simulink model "svpwmR2020a"  (Simulink 10.2)
settings: Solver=VariableStepAuto  StartTime=0.0  StopTime=0.05  RelTol=1e-3
libraries: powerlib x12, simulink x1
settings Model: Creator=Administrator  LastModifiedBy=Administrator
settings DataIOCC: SaveFormat=Dataset  SignalLoggingSaveFormat=Dataset
settings OptimizationCC: LifeSpan=auto
settings DebuggingCC: UnderspecifiedInitializationDetection=Simplified  MergeDetectMultiDrivingBlocksExec=error  FcnCallInpInsideContextMsg=error  SFUnexpectedBacktrackingDiag=error  SFNoUnconditionalDefaultTransitionDiag=error  SFExecutionAtInitializationDiag=warning
settings HardwareCC: ProdBitPerPointer=64  ProdBitPerSizeT=64  ProdBitPerPtrDiffT=64  ProdLargestAtomicFloat=Float  ProdIntDivRoundTo=Zero  ProdEndianess=LittleEndian  ProdWordSize=64  ProdHWDeviceType=Intel->x86-64 (Windows64)
settings ModelReferenceCC: PropagateSignalLabelsOutOfModel=on
settings GRTTargetCC: TargetLangStandard=C99 (ISO)  CombineOutputUpdateFcns=on  GRTInterface=off
settings ConfigComp: CovMetricSettings=dwe  CovSaveCumulativeToWorkspaceVar=off  CovSaveSingleToWorkspaceVar=off  CovExternalEMLEnable=on
settings SimscapeCC: SimscapeNormalizeSystem=off

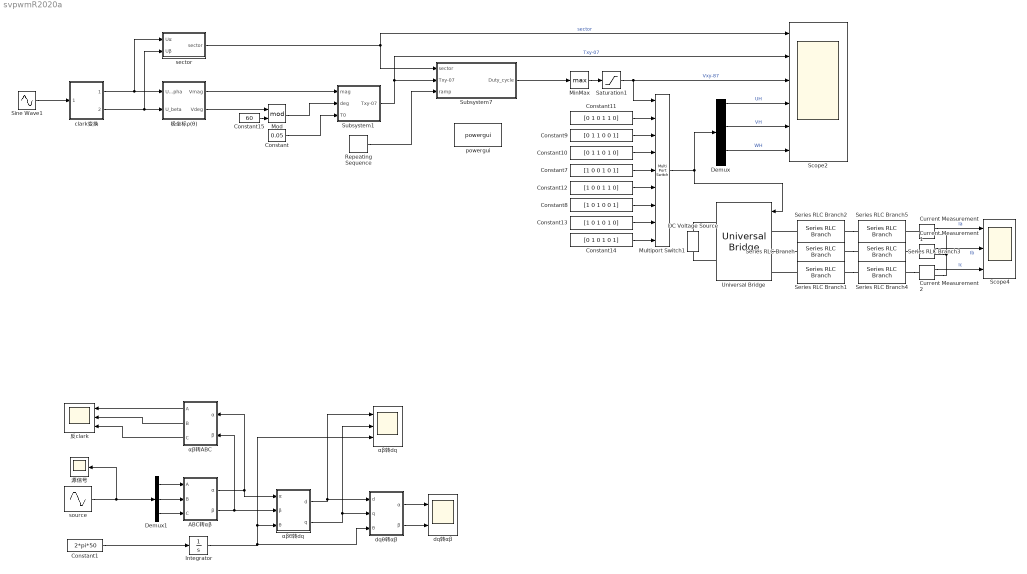
== system svpwmR2020a ==
  ABC转αβ : Subsystem
  Constant : Constant  Value=0.05
  Constant1 : Constant  Value=2*pi*50  SampleTime=1e-6
  Constant10 : Constant  Value=[0 1 1 0 1 0]  VectorParams1D=off  SampleTime=-1
  Constant11 : Constant  Value=[0 1 0 1 1 0]  VectorParams1D=off  SampleTime=-1
  Constant12 : Constant  Value=[1 0 0 1 1 0]  VectorParams1D=off  SampleTime=-1
  Constant13 : Constant  Value=[1 0 1 0 1 0]  VectorParams1D=off  SampleTime=-1
  Constant14 : Constant  Value=[0 1 0 1 0 1]  VectorParams1D=off  SampleTime=-1
  Constant15 : Constant  Value=60
  Constant7 : Constant  Value=[1 0 0 1 0 1]  VectorParams1D=off  SampleTime=-1
  Constant8 : Constant  Value=[1 0 1 0 0 1]  VectorParams1D=off  SampleTime=-1
  Constant9 : Constant  Value=[0 1 1 0 0 1]  VectorParams1D=off  SampleTime=-1
  Current Measurement : powerlib/Measurements/Current Measurement  PhasorSimulation=off  OutputType=Complex  PSBequivalent=0
  Current Measurement1 : powerlib/Measurements/Current Measurement  PhasorSimulation=off  OutputType=Complex  PSBequivalent=0
  Current Measurement2 : powerlib/Measurements/Current Measurement  PhasorSimulation=off  OutputType=Complex  PSBequivalent=0
  DC Voltage Source : powerlib/Electrical Sources/DC Voltage Source  Amplitude=100  Measurements=Voltage
  Demux : Demux  Outputs=6
  Demux1 : Demux  Outputs=3
  Integrator : Integrator
  MinMax : MinMax  Function=max
  Mod : Math  Operator=mod  SaturateOnIntegerOverflow=on
  Multiport Switch1 : MultiPortSwitch  Inputs=8
  Repeating Sequence : simulink/Sources/Repeating Sequence  rep_seq_t=[0 1e-4]  rep_seq_y=[0 1]
  Saturation1 : Saturate  UpperLimit=8  LowerLimit=1
  Scope2 : Scope  NumInputPorts=6
  Scope4 : Scope  NumInputPorts=3
  Series RLC Branch : powerlib/Elements/Series RLC Branch  LConnTagsString=__new0  RConnTagsString=__new0  BranchType=R  Resistance=2  Inductance=1e-3  SetiL0=off  InitialCurrent=0  Capacitance=1e-6  Setx0=off  InitialVoltage=0  Measurements=Branch current
  Series RLC Branch1 : powerlib/Elements/Series RLC Branch  LConnTagsString=__new0  RConnTagsString=__new0  BranchType=R  Resistance=2  Inductance=1e-3  SetiL0=off  InitialCurrent=0  Capacitance=1e-6  Setx0=off  InitialVoltage=0  Measurements=Branch current
  Series RLC Branch2 : powerlib/Elements/Series RLC Branch  LConnTagsString=__new0  RConnTagsString=__new0  BranchType=R  Resistance=2  Inductance=1e-3  SetiL0=off  InitialCurrent=0  Capacitance=1e-6  Setx0=off  InitialVoltage=0  Measurements=Branch current
  Series RLC Branch3 : powerlib/Elements/Series RLC Branch  LConnTagsString=__new0  RConnTagsString=__new0  BranchType=L  Resistance=2  Inductance=5e-3  SetiL0=off  InitialCurrent=0  Capacitance=1e-6  Setx0=off  InitialVoltage=0  Measurements=Branch current
  Series RLC Branch4 : powerlib/Elements/Series RLC Branch  LConnTagsString=__new0  RConnTagsString=__new0  BranchType=L  Resistance=2  Inductance=5e-3  SetiL0=off  InitialCurrent=0  Capacitance=1e-6  Setx0=off  InitialVoltage=0  Measurements=Branch current
  Series RLC Branch5 : powerlib/Elements/Series RLC Branch  LConnTagsString=__new0  RConnTagsString=__new0  BranchType=L  Resistance=2  Inductance=5e-3  SetiL0=off  InitialCurrent=0  Capacitance=1e-6  Setx0=off  InitialVoltage=0  Measurements=Branch current
  Sine Wave1 : Sin  Amplitude=0.5  Frequency=2*pi*50  Phase=[0 -2*pi/3 2*pi/3]  SampleTime=1e-6
  Subsystem1 : Subsystem
  Subsystem7 : Subsystem
  Universal Bridge : powerlib/Power Electronics/Universal Bridge  Arms=3  SnubberResistance=1e5  SnubberCapacitance=inf  Device=MOSFET / Diodes  Ron=1e-3  Lon=0  ForwardVoltages="[  50  50  ]"  ForwardVoltage=0  GTOparameters=[ 10e-6 , 20e-6 ]  IGBTparameters=[ 1e-6 , 2e-6 ]  Measurements=Device voltages  Measurements_2=None  converterType=Rectifier
  clark变换 : Subsystem
  dqθ转αβ : Subsystem
  dq转αβ : Scope  NumInputPorts=2
  powergui : powerlib/powergui  Priority=1  SimulationMode=Continuous  SampleTime=50e-6  frequency=60  Iterations=50  frequencyindice=0  Pbase=100e6  ErrMax=1e-4  UnitsV=kV  UnitsW=MW  buscounter=0  FunctionMessages=off  echomessages=off  EnableUseOfTLC=off  CurrentSourceSwitches=off  DisableSnubberDevices=off  DisableRonSwitches=off  DisableVfSwitches=off  DisplayEquations=off  AutomaticDiscreteSolvers=off  SolverType=Tustin/Backward Euler (TBE)  Interpol=off  ExternalGateDelay=off  methode=off  Ts=100  x0status=blocks  SPID=on  SwTol=0  HookPort=off  NonlinearTolerance=1e-4  nMaxIteration=100  ContinueOnMaxIteration=off  RestoreLinks=warning  ResistiveCurrentMeasurement=off  Frange=[0:2:500]  Ylog=off  Xlog=on  ShowGrid=off  save=off  variable=ZData  structure=0  ZoomFFT=off  StartTime=0.0  cycles=1  DisplayStyle=1  fundamental=60  FreqAxis=off  MaxFrequency=1000  frequencyindicesteady=1  RmsSteady=1  display=off
  sector : Subsystem
  source : Sin  Amplitude=100  Frequency=2*pi*50  Phase=[0 -2*pi/3 2*pi/3]  SampleTime=1e-6
  αβθ转dq : Subsystem
  αβ转ABC : Subsystem
  αβ转dq : Scope  NumInputPorts=3
  反clark : Scope  NumInputPorts=3
  极坐标ρ(θ) : Subsystem
  源信号 : Scope
  wires:
  Sine Wave1/1 -> clark变换/1(U_abc)
  极坐标ρ(θ)/2(Vdeg) -> Mod/1
  sector/1(sector) -> Scope2/1, Subsystem7/1(sector)  "sector"
  极坐标ρ(θ)/1("Vmag ") -> Subsystem1/1(mag)
  Constant/1 -> Subsystem1/3("T0 ")
  Subsystem1/1(Txy-07) -> Subsystem7/2(Txy-07), Scope2/2  "Txy-07"
  Repeating Sequence/1 -> Subsystem7/3(ramp)
  Subsystem7/1(Duty_cycle) -> MinMax/1
  MinMax/1 -> Saturation1/1
  Multiport Switch1/1 -> Demux/1, Universal Bridge/1
  Current Measurement/1 -> Scope4/1  "Ia"
  Current Measurement1/1 -> Scope4/2  "Ib"
  Current Measurement2/1 -> Scope4/3  "Ic"
  Demux/5 -> Scope2/6  "WH"
  Demux/3 -> Scope2/5  "VH"
  Demux/1 -> Scope2/4  "UH"
  Saturation1/1 -> Multiport Switch1/1, Scope2/3  "Vxy-87"
  Constant11/1 -> Multiport Switch1/2
  Constant9/1 -> Multiport Switch1/3
  Constant10/1 -> Multiport Switch1/4
  Constant7/1 -> Multiport Switch1/5
  Constant12/1 -> Multiport Switch1/6
  Constant8/1 -> Multiport Switch1/7
  Constant13/1 -> Multiport Switch1/8
  Constant14/1 -> Multiport Switch1/9
  clark变换/1(U_alpha) -> sector/1(Uα), 极坐标ρ(θ)/1("U_alpha ")
  clark变换/2(U_beta) -> sector/2(Uβ), 极坐标ρ(θ)/2(U_beta)
  Constant15/1 -> Mod/2
  Mod/1 -> Subsystem1/2(deg)
  Demux1/1 -> ABC转αβ/1(A)
  Demux1/3 -> ABC转αβ/3(C)
  Demux1/2 -> ABC转αβ/2(B)
  Constant1/1 -> Integrator/1
  source/1 -> Demux1/1, 源信号/1
  αβθ转dq/1(d) -> dqθ转αβ/1(d), αβ转dq/1
  Integrator/1 -> dqθ转αβ/3(θ), αβθ转dq/3(θ), αβ转dq/3
  αβθ转dq/2(q) -> αβ转dq/2, dqθ转αβ/2(q)
  αβ转ABC/2(B) -> 反clark/2
  αβ转ABC/1(A) -> 反clark/1
  αβ转ABC/3(C) -> 反clark/3
  ABC转αβ/2(β) -> αβ转ABC/2(β), αβθ转dq/2(β)
  ABC转αβ/1(α) -> αβ转ABC/1(α), αβθ转dq/1(α)
  dqθ转αβ/1(α) -> dq转αβ/1
  dqθ转αβ/2(β) -> dq转αβ/2
  connections:
  DC Voltage Source/RConn1 -- Universal Bridge/RConn1
  DC Voltage Source/LConn1 -- Universal Bridge/RConn2
  Series RLC Branch1/LConn1 -- Universal Bridge/LConn3
  Universal Bridge/LConn2 -- Series RLC Branch/LConn1
  Series RLC Branch2/LConn1 -- Universal Bridge/LConn1
  Series RLC Branch2/RConn1 -- Series RLC Branch5/LConn1
  Series RLC Branch/RConn1 -- Series RLC Branch3/LConn1
  Series RLC Branch1/RConn1 -- Series RLC Branch4/LConn1
  Current Measurement/LConn1 -- Series RLC Branch5/RConn1
  Series RLC Branch4/RConn1 -- Current Measurement2/LConn1
  Series RLC Branch3/RConn1 -- Current Measurement1/LConn1
  Current Measurement2/RConn1 -- Current Measurement1/RConn1 -- Current Measurement/RConn1

== system svpwmR2020a/ABC转αβ ==
  A : Inport
  B : Inport  Port=2
  C : Inport  Port=3
  Fcn : Fcn  Expr=2/3*(sqrt(3)/2*u(2)-sqrt(3)/2*u(3))
  Fcn1 : Fcn  Expr=2/3*(u(1)-0.5*u(2)-0.5*u(3))
  Mux : Mux  Inputs=3
  α : Outport
  β : Outport  Port=2
  wires:
  Mux/1 -> Fcn/1, Fcn1/1
  Fcn/1 -> β/1
  Fcn1/1 -> α/1
  A/1 -> Mux/1
  B/1 -> Mux/2
  C/1 -> Mux/3

== system svpwmR2020a/Subsystem1 ==
  mag : Inport
  deg : Inport  Port=2
  "T0 " : Inport  Port=3
  Mux : Mux
  duty-cycles : Subsystem
  Txy-07 : Outport
  wires:
  duty-cycles/2(Ty) -> Mux/2
  duty-cycles/4(T7) -> Mux/4
  duty-cycles/1(Tx) -> Mux/1
  deg/1 -> duty-cycles/2(deg)
  "T0 "/1 -> duty-cycles/3("T0 ")
  Mux/1 -> Txy-07/1
  duty-cycles/3(T0) -> Mux/3
  mag/1 -> duty-cycles/1(mag)

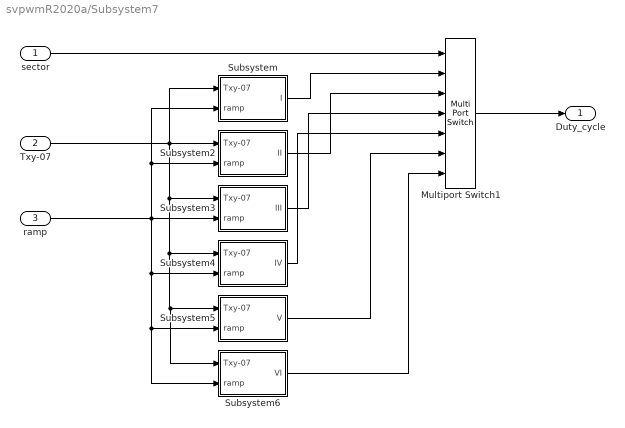
== system svpwmR2020a/Subsystem7 ==
  sector : Inport
  Txy-07 : Inport  Port=2
  ramp : Inport  Port=3
  Multiport Switch1 : MultiPortSwitch  Inputs=6
  Subsystem : Subsystem
  Subsystem2 : Subsystem
  Subsystem3 : Subsystem
  Subsystem4 : Subsystem
  Subsystem5 : Subsystem
  Subsystem6 : Subsystem
  Duty_cycle : Outport
  wires:
  Txy-07/1 -> Subsystem/1(Txy-07), Subsystem2/1(Txy-07), Subsystem3/1(Txy-07), Subsystem4/1(Txy-07), Subsystem6/1(Txy-07), Subsystem5/1(Txy-07)
  ramp/1 -> Subsystem3/2(ramp), Subsystem/2(ramp), Subsystem2/2(ramp), Subsystem5/2(ramp), Subsystem6/2(ramp), Subsystem4/2(ramp)
  Subsystem/1(I) -> Multiport Switch1/2
  Subsystem6/1(VI) -> Multiport Switch1/7
  Subsystem5/1(V) -> Multiport Switch1/6
  Subsystem3/1(III) -> Multiport Switch1/4
  Multiport Switch1/1 -> Duty_cycle/1
  Subsystem2/1(II) -> Multiport Switch1/3
  Subsystem4/1(IV) -> Multiport Switch1/5
  sector/1 -> Multiport Switch1/1

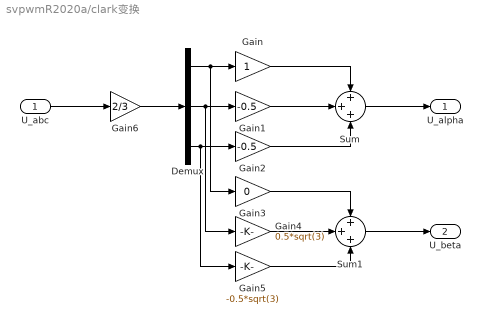
== system svpwmR2020a/clark变换 ==
  U_abc : Inport
  Demux : Demux  Outputs=3
  Gain : Gain
  Gain1 : Gain  Gain=-0.5
  Gain2 : Gain  Gain=-0.5
  Gain3 : Gain  Gain=0
  Gain4 : Gain  Gain=0.5*sqrt(3)
  Gain5 : Gain  Gain=-0.5*sqrt(3)
  Gain6 : Gain  Gain=2/3
  Sum : Sum  Inputs=+++
  Sum1 : Sum  Inputs=+++
  U_alpha : Outport
  U_beta : Outport  Port=2
  wires:
  Gain5/1 -> Sum1/3
  Gain4/1 -> Sum1/2
  Gain1/1 -> Sum/2
  Gain2/1 -> Sum/3
  Demux/1 -> Gain/1, Gain3/1
  Sum/1 -> U_alpha/1
  Sum1/1 -> U_beta/1
  Demux/3 -> Gain5/1, Gain2/1
  Gain/1 -> Sum/1
  Demux/2 -> Gain4/1, Gain1/1
  Gain3/1 -> Sum1/1
  U_abc/1 -> Gain6/1
  Gain6/1 -> Demux/1

== system svpwmR2020a/dqθ转αβ ==
  d : Inport
  q : Inport  Port=2
  θ : Inport  Port=3
  Fcn : Fcn  Expr=u(1)*sin(u(3))+u(2)*cos(u(3))
  Fcn1 : Fcn  Expr=u(1)*cos(u(3))-u(2)*sin(u(3))
  Mux : Mux  Inputs=3
  α : Outport
  β : Outport  Port=2
  wires:
  θ/1 -> Mux/3
  d/1 -> Mux/1
  Fcn1/1 -> α/1
  Fcn/1 -> β/1
  Mux/1 -> Fcn1/1, Fcn/1
  q/1 -> Mux/2

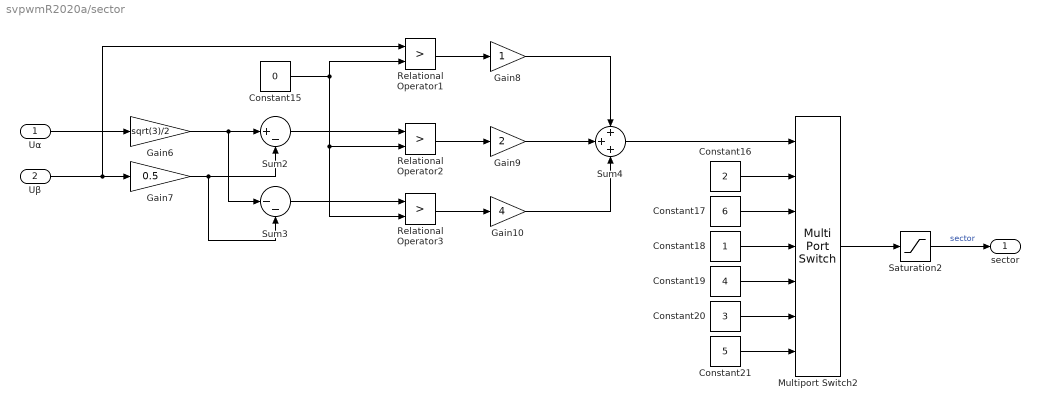
== system svpwmR2020a/sector ==
  Uα : Inport
  Uβ : Inport  Port=2
  Constant15 : Constant  Value=0
  Constant16 : Constant  Value=2
  Constant17 : Constant  Value=6
  Constant18 : Constant
  Constant19 : Constant  Value=4
  Constant20 : Constant  Value=3
  Constant21 : Constant  Value=5
  Gain10 : Gain  Gain=4
  Gain6 : Gain  Gain=sqrt(3)/2
  Gain7 : Gain  Gain=0.5
  Gain8 : Gain
  Gain9 : Gain  Gain=2
  Multiport Switch2 : MultiPortSwitch  Inputs=6
  Relational Operator1 : RelationalOperator  Operator=>  OutDataTypeStr=boolean  RndMeth=Simplest
  Relational Operator2 : RelationalOperator  Operator=>  OutDataTypeStr=boolean  RndMeth=Simplest
  Relational Operator3 : RelationalOperator  Operator=>  OutDataTypeStr=boolean  RndMeth=Simplest
  Saturation2 : Saturate  UpperLimit=6  LowerLimit=1
  Sum2 : Sum  Inputs=|+-
  Sum3 : Sum  Inputs=|--
  Sum4 : Sum  Inputs=+++
  sector : Outport
  wires:
  Relational Operator1/1 -> Gain8/1
  Sum3/1 -> Relational Operator3/1
  Gain6/1 -> Sum3/1, Sum2/1
  Constant15/1 -> Relational Operator1/2, Relational Operator3/2, Relational Operator2/2
  Gain9/1 -> Sum4/2
  Uβ/1 -> Relational Operator1/1, Gain7/1
  Relational Operator3/1 -> Gain10/1
  Relational Operator2/1 -> Gain9/1
  Constant17/1 -> Multiport Switch2/3
  Constant16/1 -> Multiport Switch2/2
  Constant21/1 -> Multiport Switch2/7
  Gain10/1 -> Sum4/3
  Gain7/1 -> Sum2/2, Sum3/2
  Sum2/1 -> Relational Operator2/1
  Uα/1 -> Gain6/1
  Constant18/1 -> Multiport Switch2/4
  Constant19/1 -> Multiport Switch2/5
  Constant20/1 -> Multiport Switch2/6
  Gain8/1 -> Sum4/1
  Sum4/1 -> Multiport Switch2/1
  Multiport Switch2/1 -> Saturation2/1
  Saturation2/1 -> sector/1  "sector"

== system svpwmR2020a/αβθ转dq ==
  α : Inport
  β : Inport  Port=2
  θ : Inport  Port=3
  Fcn : Fcn  Expr=-u(1)*sin(u(3))+u(2)*cos(u(3))
  Fcn1 : Fcn  Expr=u(1)*cos(u(3))+u(2)*sin(u(3))
  Gain : Gain
  Mux : Mux  Inputs=3
  d : Outport
  q : Outport  Port=2
  wires:
  θ/1 -> Mux/3
  β/1 -> Mux/2
  α/1 -> Mux/1
  Fcn1/1 -> d/1
  Mux/1 -> Fcn1/1, Fcn/1
  Fcn/1 -> Gain/1
  Gain/1 -> q/1

== system svpwmR2020a/αβ转ABC ==
  α : Inport
  β : Inport  Port=2
  Fcn : Fcn  Expr=-0.5*u(1)+sqrt(3)/2*u(2)
  Fcn1 : Fcn  Expr=u(1)
  Fcn2 : Fcn  Expr=-0.5*u(1)-sqrt(3)/2*u(2)
  Mux : Mux  Inputs=2
  A : Outport
  B : Outport  Port=2
  C : Outport  Port=3
  wires:
  β/1 -> Mux/2
  α/1 -> Mux/1
  Fcn1/1 -> A/1
  Fcn/1 -> B/1
  Mux/1 -> Fcn1/1, Fcn2/1, Fcn/1
  Fcn2/1 -> C/1

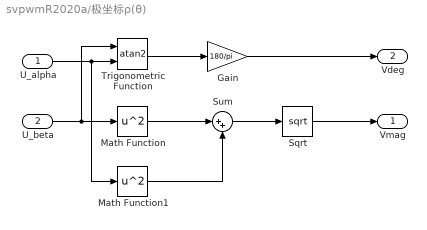
== system svpwmR2020a/极坐标ρ(θ) ==
  "U_alpha " : Inport
  U_beta : Inport  Port=2
  Gain : Gain  Gain=180/pi
  Math Function : Math  Operator=square  SignedPower=on  SaturateOnIntegerOverflow=on
  Math Function1 : Math  Operator=square  SignedPower=on  SaturateOnIntegerOverflow=on
  Sqrt : Sqrt  SaturateOnIntegerOverflow=on
  Sum : Sum  Inputs=|++
  Trigonometric Function : Trigonometry  Operator=atan2
  "Vmag " : Outport
  Vdeg : Outport  Port=2
  wires:
  "U_alpha "/1 -> Math Function1/1, Trigonometric Function/2
  U_beta/1 -> Trigonometric Function/1, Math Function/1
  Math Function/1 -> Sum/1
  Math Function1/1 -> Sum/2
  Sum/1 -> Sqrt/1
  Gain/1 -> Vdeg/1
  Trigonometric Function/1 -> Gain/1
  Sqrt/1 -> "Vmag "/1

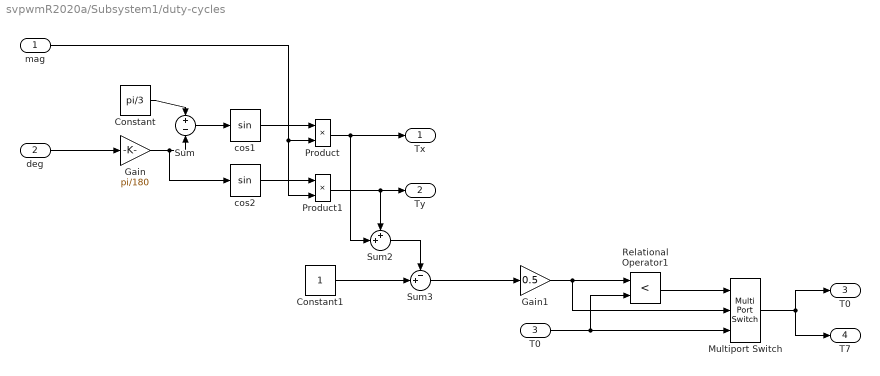
== system svpwmR2020a/Subsystem1/duty-cycles ==
  mag : Inport
  deg : Inport  Port=2
  "T0 " : Inport  Port=3
  Constant : Constant  Value=pi/3
  Constant1 : Constant
  Gain : Gain  Gain=pi/180
  Gain1 : Gain  Gain=0.5
  Multiport Switch : MultiPortSwitch  DataPortOrder=Zero-based contiguous  Inputs=2  zeroidx=on
  Product : Product
  Product1 : Product
  Relational Operator1 : RelationalOperator  Operator=<  OutDataTypeStr=boolean  RndMeth=Simplest
  Sum : Sum  Inputs=+|-
  Sum2 : Sum  Inputs=++|
  Sum3 : Sum  Inputs=-+|
  cos1 : Trigonometry
  cos2 : Trigonometry
  Tx : Outport
  Ty : Outport  Port=2
  T0 : Outport  Port=3
  T7 : Outport  Port=4
  wires:
  Gain/1 -> cos2/1, Sum/2
  cos1/1 -> Product/1
  Sum/1 -> cos1/1
  mag/1 -> Product1/2, Product/2
  deg/1 -> Gain/1
  Product1/1 -> Sum2/1, Ty/1
  Product/1 -> Sum2/2, Tx/1
  cos2/1 -> Product1/1
  Constant/1 -> Sum/1
  Sum2/1 -> Sum3/1
  Constant1/1 -> Sum3/2
  Sum3/1 -> Gain1/1
  Gain1/1 -> Multiport Switch/2, Relational Operator1/1
  "T0 "/1 -> Relational Operator1/2, Multiport Switch/3
  Relational Operator1/1 -> Multiport Switch/1
  Multiport Switch/1 -> T7/1, T0/1

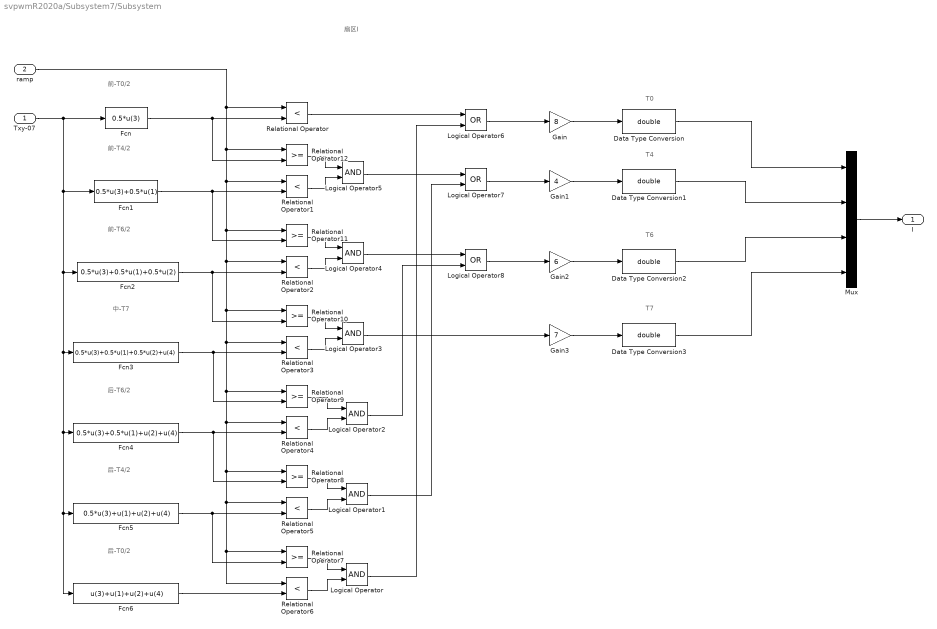
== system svpwmR2020a/Subsystem7/Subsystem ==
  note: 扇区I
  note: 前-T0/2
  note: 前-T4/2
  note: 前-T6/2
  note: 中-T7
  note: 后-T6/2
  note: 后-T4/2
  note: 后-T0/2
  note: T0
  note: T4
  note: T6
  note: T7
  Txy-07 : Inport
  ramp : Inport  Port=2
  Data Type Conversion{,1..3} (4 alike) : DataTypeConversion  OutDataTypeStr=double
  Fcn : Fcn  Expr=0.5*u(3)
  Fcn1 : Fcn  Expr=0.5*u(3)+0.5*u(1)
  Fcn2 : Fcn  Expr=0.5*u(3)+0.5*u(1)+0.5*u(2)
  Fcn3 : Fcn  Expr=0.5*u(3)+0.5*u(1)+0.5*u(2)+u(4)
  Fcn4 : Fcn  Expr=0.5*u(3)+0.5*u(1)+u(2)+u(4)
  Fcn5 : Fcn  Expr=0.5*u(3)+u(1)+u(2)+u(4)
  Fcn6 : Fcn  Expr=u(3)+u(1)+u(2)+u(4)
  Gain : Gain  Gain=8
  Gain1 : Gain  Gain=4
  Gain2 : Gain  Gain=6
  Gain3 : Gain  Gain=7
  Logical Operator{,1..5} (6 alike) : Logic  AllPortsSameDT=off  OutDataTypeStr=boolean
  Logical Operator6 : Logic  Operator=OR  AllPortsSameDT=off  OutDataTypeStr=boolean
  Logical Operator7 : Logic  Operator=OR  AllPortsSameDT=off  OutDataTypeStr=boolean
  Logical Operator8 : Logic  Operator=OR  AllPortsSameDT=off  OutDataTypeStr=boolean
  Mux : Mux
  Relational Operator{,1..6} (7 alike) : RelationalOperator  Operator=<  OutDataTypeStr=boolean  RndMeth=Simplest
  Relational Operator{7..12} (6 alike) : RelationalOperator  OutDataTypeStr=boolean  RndMeth=Simplest
  I : Outport
  wires:
  Txy-07/1 -> Fcn/1, Fcn1/1, Fcn2/1, Fcn6/1, Fcn5/1, Fcn4/1, Fcn3/1
  Fcn/1 -> Relational Operator12/2, Relational Operator/2
  Fcn1/1 -> Relational Operator11/2, Relational Operator1/2
  Fcn2/1 -> Relational Operator10/2, Relational Operator2/2
  Fcn3/1 -> Relational Operator9/2, Relational Operator3/2
  Fcn4/1 -> Relational Operator8/2, Relational Operator4/2
  Fcn6/1 -> Relational Operator6/2
  Fcn5/1 -> Relational Operator7/2, Relational Operator5/2
  Relational Operator7/1 -> Logical Operator/1
  Relational Operator6/1 -> Logical Operator/2
  Relational Operator12/1 -> Logical Operator5/1
  Relational Operator1/1 -> Logical Operator5/2
  Relational Operator11/1 -> Logical Operator4/1
  Relational Operator2/1 -> Logical Operator4/2
  Relational Operator10/1 -> Logical Operator3/1
  Relational Operator3/1 -> Logical Operator3/2
  Relational Operator9/1 -> Logical Operator2/1
  Relational Operator4/1 -> Logical Operator2/2
  Relational Operator8/1 -> Logical Operator1/1
  Relational Operator5/1 -> Logical Operator1/2
  ramp/1 -> Relational Operator12/1, Relational Operator11/1, Relational Operator10/1, Relational Operator9/1, Relational Operator8/1, Relational Operator7/1, Relational Operator6/1, Relational Operator5/1, Relational Operator4/1, Relational Operator3/1, Relational Operator2/1, Relational Operator1/1, Relational Operator/1
  Relational Operator/1 -> Logical Operator6/1
  Logical Operator/1 -> Logical Operator6/2
  Logical Operator5/1 -> Logical Operator7/1
  Logical Operator1/1 -> Logical Operator7/2
  Logical Operator4/1 -> Logical Operator8/1
  Logical Operator2/1 -> Logical Operator8/2
  Logical Operator6/1 -> Gain/1
  Logical Operator7/1 -> Gain1/1
  Logical Operator8/1 -> Gain2/1
  Logical Operator3/1 -> Gain3/1
  Gain3/1 -> Data Type Conversion3/1
  Gain2/1 -> Data Type Conversion2/1
  Gain1/1 -> Data Type Conversion1/1
  Gain/1 -> Data Type Conversion/1
  Data Type Conversion/1 -> Mux/1
  Data Type Conversion1/1 -> Mux/2
  Data Type Conversion2/1 -> Mux/3
  Data Type Conversion3/1 -> Mux/4
  Mux/1 -> I/1

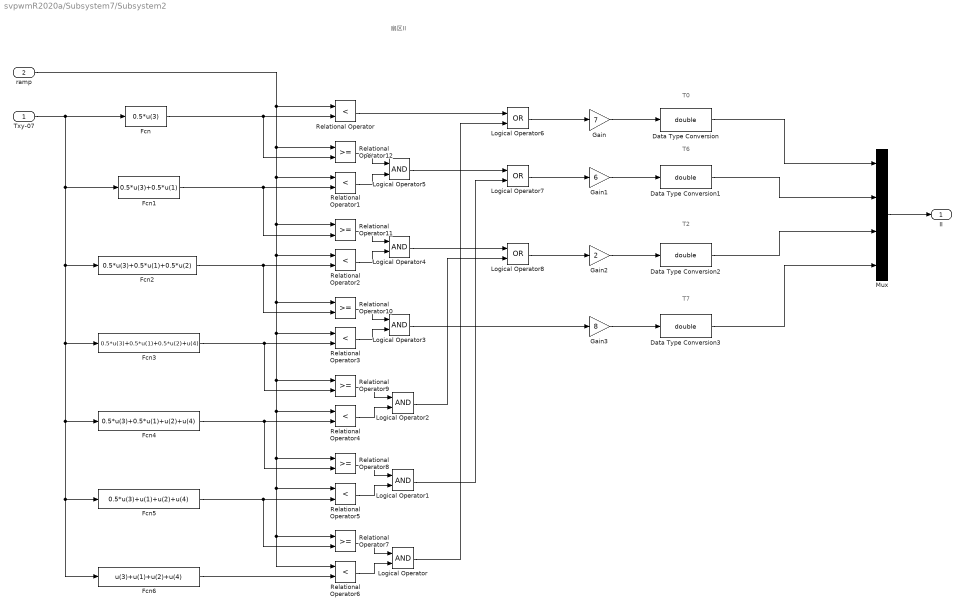
== system svpwmR2020a/Subsystem7/Subsystem2 ==
  note: T0
  note: 扇区II
  note: T2
  note: T7
  note: T6
  Txy-07 : Inport
  ramp : Inport  Port=2
  Data Type Conversion{,1..3} (4 alike) : DataTypeConversion  OutDataTypeStr=double
  Fcn : Fcn  Expr=0.5*u(3)
  Fcn1 : Fcn  Expr=0.5*u(3)+0.5*u(1)
  Fcn2 : Fcn  Expr=0.5*u(3)+0.5*u(1)+0.5*u(2)
  Fcn3 : Fcn  Expr=0.5*u(3)+0.5*u(1)+0.5*u(2)+u(4)
  Fcn4 : Fcn  Expr=0.5*u(3)+0.5*u(1)+u(2)+u(4)
  Fcn5 : Fcn  Expr=0.5*u(3)+u(1)+u(2)+u(4)
  Fcn6 : Fcn  Expr=u(3)+u(1)+u(2)+u(4)
  Gain : Gain  Gain=7
  Gain1 : Gain  Gain=6
  Gain2 : Gain  Gain=2
  Gain3 : Gain  Gain=8
  Logical Operator{,1..5} (6 alike) : Logic  AllPortsSameDT=off  OutDataTypeStr=boolean
  Logical Operator6 : Logic  Operator=OR  AllPortsSameDT=off  OutDataTypeStr=boolean
  Logical Operator7 : Logic  Operator=OR  AllPortsSameDT=off  OutDataTypeStr=boolean
  Logical Operator8 : Logic  Operator=OR  AllPortsSameDT=off  OutDataTypeStr=boolean
  Mux : Mux
  Relational Operator{,1..6} (7 alike) : RelationalOperator  Operator=<  OutDataTypeStr=boolean  RndMeth=Simplest
  Relational Operator{7..12} (6 alike) : RelationalOperator  OutDataTypeStr=boolean  RndMeth=Simplest
  II : Outport
  wires:
  Mux/1 -> II/1
  Data Type Conversion3/1 -> Mux/4
  Data Type Conversion2/1 -> Mux/3
  Data Type Conversion1/1 -> Mux/2
  Data Type Conversion/1 -> Mux/1
  Gain/1 -> Data Type Conversion/1
  Gain1/1 -> Data Type Conversion1/1
  Gain2/1 -> Data Type Conversion2/1
  Gain3/1 -> Data Type Conversion3/1
  Logical Operator3/1 -> Gain3/1
  Logical Operator8/1 -> Gain2/1
  Logical Operator7/1 -> Gain1/1
  Logical Operator6/1 -> Gain/1
  Logical Operator2/1 -> Logical Operator8/2
  Logical Operator4/1 -> Logical Operator8/1
  Logical Operator1/1 -> Logical Operator7/2
  Logical Operator5/1 -> Logical Operator7/1
  Logical Operator/1 -> Logical Operator6/2
  Relational Operator/1 -> Logical Operator6/1
  ramp/1 -> Relational Operator/1, Relational Operator1/1, Relational Operator2/1, Relational Operator3/1, Relational Operator4/1, Relational Operator5/1, Relational Operator6/1, Relational Operator7/1, Relational Operator8/1, Relational Operator9/1, Relational Operator10/1, Relational Operator11/1, Relational Operator12/1
  Relational Operator5/1 -> Logical Operator1/2
  Relational Operator8/1 -> Logical Operator1/1
  Relational Operator4/1 -> Logical Operator2/2
  Relational Operator9/1 -> Logical Operator2/1
  Relational Operator3/1 -> Logical Operator3/2
  Relational Operator10/1 -> Logical Operator3/1
  Relational Operator2/1 -> Logical Operator4/2
  Relational Operator11/1 -> Logical Operator4/1
  Relational Operator1/1 -> Logical Operator5/2
  Relational Operator12/1 -> Logical Operator5/1
  Relational Operator6/1 -> Logical Operator/2
  Relational Operator7/1 -> Logical Operator/1
  Fcn5/1 -> Relational Operator5/2, Relational Operator7/2
  Fcn6/1 -> Relational Operator6/2
  Fcn4/1 -> Relational Operator4/2, Relational Operator8/2
  Fcn3/1 -> Relational Operator3/2, Relational Operator9/2
  Fcn2/1 -> Relational Operator2/2, Relational Operator10/2
  Fcn1/1 -> Relational Operator1/2, Relational Operator11/2
  Fcn/1 -> Relational Operator/2, Relational Operator12/2
  Txy-07/1 -> Fcn/1, Fcn2/1, Fcn3/1, Fcn4/1, Fcn6/1, Fcn5/1, Fcn1/1

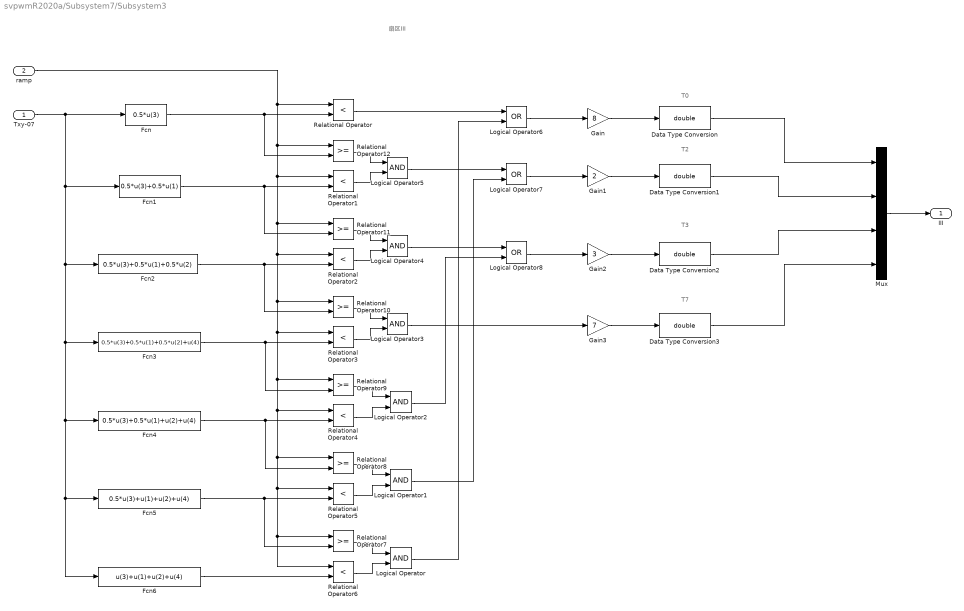
== system svpwmR2020a/Subsystem7/Subsystem3 ==
  note: T7
  note: 扇区III
  note: T0
  note: T2
  note: T3
  Txy-07 : Inport
  ramp : Inport  Port=2
  Data Type Conversion{,1..3} (4 alike) : DataTypeConversion  OutDataTypeStr=double
  Fcn : Fcn  Expr=0.5*u(3)
  Fcn1 : Fcn  Expr=0.5*u(3)+0.5*u(1)
  Fcn2 : Fcn  Expr=0.5*u(3)+0.5*u(1)+0.5*u(2)
  Fcn3 : Fcn  Expr=0.5*u(3)+0.5*u(1)+0.5*u(2)+u(4)
  Fcn4 : Fcn  Expr=0.5*u(3)+0.5*u(1)+u(2)+u(4)
  Fcn5 : Fcn  Expr=0.5*u(3)+u(1)+u(2)+u(4)
  Fcn6 : Fcn  Expr=u(3)+u(1)+u(2)+u(4)
  Gain : Gain  Gain=8
  Gain1 : Gain  Gain=2
  Gain2 : Gain  Gain=3
  Gain3 : Gain  Gain=7
  Logical Operator{,1..5} (6 alike) : Logic  AllPortsSameDT=off  OutDataTypeStr=boolean
  Logical Operator6 : Logic  Operator=OR  AllPortsSameDT=off  OutDataTypeStr=boolean
  Logical Operator7 : Logic  Operator=OR  AllPortsSameDT=off  OutDataTypeStr=boolean
  Logical Operator8 : Logic  Operator=OR  AllPortsSameDT=off  OutDataTypeStr=boolean
  Mux : Mux
  Relational Operator{,1..6} (7 alike) : RelationalOperator  Operator=<  OutDataTypeStr=boolean  RndMeth=Simplest
  Relational Operator{7..12} (6 alike) : RelationalOperator  OutDataTypeStr=boolean  RndMeth=Simplest
  III : Outport
  wires:
  Relational Operator7/1 -> Logical Operator/1
  Relational Operator6/1 -> Logical Operator/2
  Relational Operator12/1 -> Logical Operator5/1
  Relational Operator1/1 -> Logical Operator5/2
  Relational Operator11/1 -> Logical Operator4/1
  Relational Operator2/1 -> Logical Operator4/2
  Relational Operator10/1 -> Logical Operator3/1
  Relational Operator3/1 -> Logical Operator3/2
  Relational Operator9/1 -> Logical Operator2/1
  Relational Operator4/1 -> Logical Operator2/2
  Relational Operator8/1 -> Logical Operator1/1
  Relational Operator5/1 -> Logical Operator1/2
  Relational Operator/1 -> Logical Operator6/1
  Logical Operator/1 -> Logical Operator6/2
  Logical Operator5/1 -> Logical Operator7/1
  Logical Operator1/1 -> Logical Operator7/2
  Logical Operator4/1 -> Logical Operator8/1
  Logical Operator2/1 -> Logical Operator8/2
  Logical Operator6/1 -> Gain/1
  Logical Operator7/1 -> Gain1/1
  Logical Operator8/1 -> Gain2/1
  Logical Operator3/1 -> Gain3/1
  Gain3/1 -> Data Type Conversion3/1
  Gain2/1 -> Data Type Conversion2/1
  Gain1/1 -> Data Type Conversion1/1
  Gain/1 -> Data Type Conversion/1
  Data Type Conversion/1 -> Mux/1
  Data Type Conversion1/1 -> Mux/2
  Data Type Conversion2/1 -> Mux/3
  Data Type Conversion3/1 -> Mux/4
  Mux/1 -> III/1
  Fcn1/1 -> Relational Operator1/2, Relational Operator11/2
  Fcn3/1 -> Relational Operator9/2, Relational Operator3/2
  ramp/1 -> Relational Operator/1, Relational Operator12/1, Relational Operator1/1, Relational Operator11/1, Relational Operator2/1, Relational Operator10/1, Relational Operator3/1, Relational Operator9/1, Relational Operator4/1, Relational Operator8/1, Relational Operator5/1, Relational Operator7/1, Relational Operator6/1
  Fcn6/1 -> Relational Operator6/2
  Txy-07/1 -> Fcn/1, Fcn2/1, Fcn3/1, Fcn4/1, Fcn6/1, Fcn5/1, Fcn1/1
  Fcn2/1 -> Relational Operator10/2, Relational Operator2/2
  Fcn5/1 -> Relational Operator7/2, Relational Operator5/2
  Fcn4/1 -> Relational Operator4/2, Relational Operator8/2
  Fcn/1 -> Relational Operator12/2, Relational Operator/2

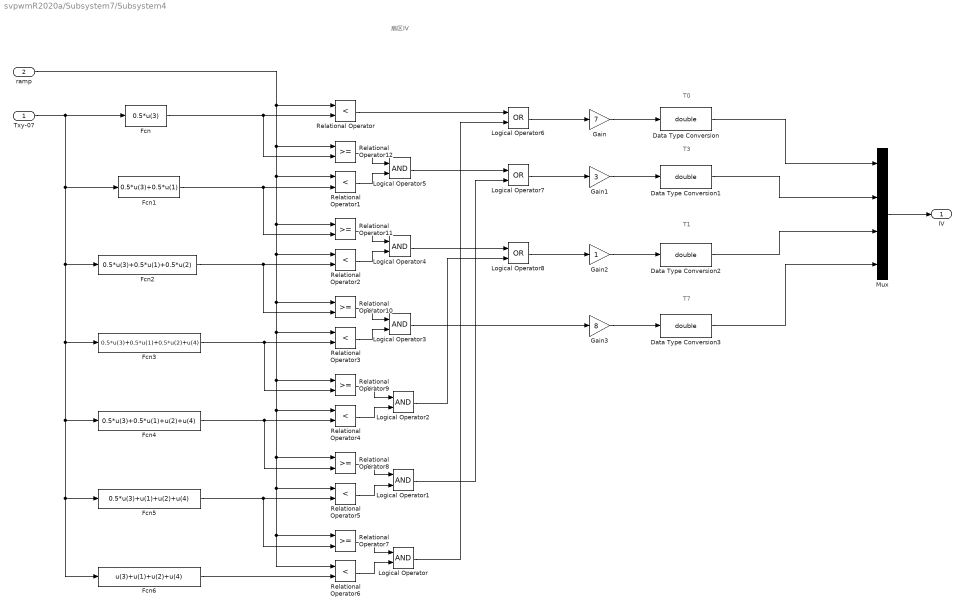
== system svpwmR2020a/Subsystem7/Subsystem4 ==
  note: T7
  note: 扇区IV
  note: T0
  note: T3
  note: T1
  Txy-07 : Inport
  ramp : Inport  Port=2
  Data Type Conversion{,1..3} (4 alike) : DataTypeConversion  OutDataTypeStr=double
  Fcn : Fcn  Expr=0.5*u(3)
  Fcn1 : Fcn  Expr=0.5*u(3)+0.5*u(1)
  Fcn2 : Fcn  Expr=0.5*u(3)+0.5*u(1)+0.5*u(2)
  Fcn3 : Fcn  Expr=0.5*u(3)+0.5*u(1)+0.5*u(2)+u(4)
  Fcn4 : Fcn  Expr=0.5*u(3)+0.5*u(1)+u(2)+u(4)
  Fcn5 : Fcn  Expr=0.5*u(3)+u(1)+u(2)+u(4)
  Fcn6 : Fcn  Expr=u(3)+u(1)+u(2)+u(4)
  Gain : Gain  Gain=7
  Gain1 : Gain  Gain=3
  Gain2 : Gain
  Gain3 : Gain  Gain=8
  Logical Operator{,1..5} (6 alike) : Logic  AllPortsSameDT=off  OutDataTypeStr=boolean
  Logical Operator6 : Logic  Operator=OR  AllPortsSameDT=off  OutDataTypeStr=boolean
  Logical Operator7 : Logic  Operator=OR  AllPortsSameDT=off  OutDataTypeStr=boolean
  Logical Operator8 : Logic  Operator=OR  AllPortsSameDT=off  OutDataTypeStr=boolean
  Mux : Mux
  Relational Operator{,1..6} (7 alike) : RelationalOperator  Operator=<  OutDataTypeStr=boolean  RndMeth=Simplest
  Relational Operator{7..12} (6 alike) : RelationalOperator  OutDataTypeStr=boolean  RndMeth=Simplest
  IV : Outport
  wires:
  Mux/1 -> IV/1
  Data Type Conversion3/1 -> Mux/4
  Data Type Conversion2/1 -> Mux/3
  Data Type Conversion1/1 -> Mux/2
  Data Type Conversion/1 -> Mux/1
  Gain/1 -> Data Type Conversion/1
  Gain1/1 -> Data Type Conversion1/1
  Gain2/1 -> Data Type Conversion2/1
  Gain3/1 -> Data Type Conversion3/1
  Logical Operator3/1 -> Gain3/1
  Logical Operator8/1 -> Gain2/1
  Logical Operator7/1 -> Gain1/1
  Logical Operator6/1 -> Gain/1
  Logical Operator2/1 -> Logical Operator8/2
  Logical Operator4/1 -> Logical Operator8/1
  Logical Operator1/1 -> Logical Operator7/2
  Logical Operator5/1 -> Logical Operator7/1
  Logical Operator/1 -> Logical Operator6/2
  Relational Operator/1 -> Logical Operator6/1
  Relational Operator5/1 -> Logical Operator1/2
  Relational Operator8/1 -> Logical Operator1/1
  Relational Operator4/1 -> Logical Operator2/2
  Relational Operator9/1 -> Logical Operator2/1
  Relational Operator3/1 -> Logical Operator3/2
  Relational Operator10/1 -> Logical Operator3/1
  Relational Operator2/1 -> Logical Operator4/2
  Relational Operator11/1 -> Logical Operator4/1
  Relational Operator1/1 -> Logical Operator5/2
  Relational Operator12/1 -> Logical Operator5/1
  Relational Operator6/1 -> Logical Operator/2
  Relational Operator7/1 -> Logical Operator/1
  Fcn1/1 -> Relational Operator11/2, Relational Operator1/2
  Fcn3/1 -> Relational Operator3/2, Relational Operator9/2
  ramp/1 -> Relational Operator/1, Relational Operator12/1, Relational Operator1/1, Relational Operator11/1, Relational Operator2/1, Relational Operator10/1, Relational Operator3/1, Relational Operator9/1, Relational Operator4/1, Relational Operator8/1, Relational Operator5/1, Relational Operator6/1, Relational Operator7/1
  Fcn6/1 -> Relational Operator6/2
  Txy-07/1 -> Fcn/1, Fcn2/1, Fcn3/1, Fcn4/1, Fcn6/1, Fcn5/1, Fcn1/1
  Fcn2/1 -> Relational Operator10/2, Relational Operator2/2
  Fcn5/1 -> Relational Operator5/2, Relational Operator7/2
  Fcn4/1 -> Relational Operator4/2, Relational Operator8/2
  Fcn/1 -> Relational Operator12/2, Relational Operator/2

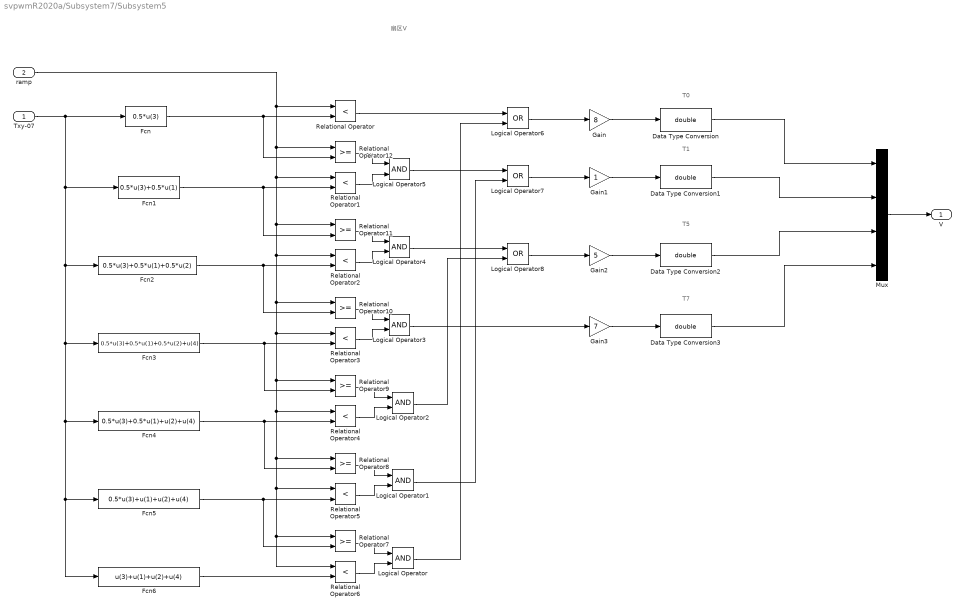
== system svpwmR2020a/Subsystem7/Subsystem5 ==
  note: T7
  note: 扇区V
  note: T0
  note: T1
  note: T5
  Txy-07 : Inport
  ramp : Inport  Port=2
  Data Type Conversion{,1..3} (4 alike) : DataTypeConversion  OutDataTypeStr=double
  Fcn : Fcn  Expr=0.5*u(3)
  Fcn1 : Fcn  Expr=0.5*u(3)+0.5*u(1)
  Fcn2 : Fcn  Expr=0.5*u(3)+0.5*u(1)+0.5*u(2)
  Fcn3 : Fcn  Expr=0.5*u(3)+0.5*u(1)+0.5*u(2)+u(4)
  Fcn4 : Fcn  Expr=0.5*u(3)+0.5*u(1)+u(2)+u(4)
  Fcn5 : Fcn  Expr=0.5*u(3)+u(1)+u(2)+u(4)
  Fcn6 : Fcn  Expr=u(3)+u(1)+u(2)+u(4)
  Gain : Gain  Gain=8
  Gain1 : Gain
  Gain2 : Gain  Gain=5
  Gain3 : Gain  Gain=7
  Logical Operator{,1..5} (6 alike) : Logic  AllPortsSameDT=off  OutDataTypeStr=boolean
  Logical Operator6 : Logic  Operator=OR  AllPortsSameDT=off  OutDataTypeStr=boolean
  Logical Operator7 : Logic  Operator=OR  AllPortsSameDT=off  OutDataTypeStr=boolean
  Logical Operator8 : Logic  Operator=OR  AllPortsSameDT=off  OutDataTypeStr=boolean
  Mux : Mux
  Relational Operator{,1..6} (7 alike) : RelationalOperator  Operator=<  OutDataTypeStr=boolean  RndMeth=Simplest
  Relational Operator{7..12} (6 alike) : RelationalOperator  OutDataTypeStr=boolean  RndMeth=Simplest
  V : Outport
  wires:
  Relational Operator7/1 -> Logical Operator/1
  Relational Operator6/1 -> Logical Operator/2
  Relational Operator12/1 -> Logical Operator5/1
  Relational Operator1/1 -> Logical Operator5/2
  Relational Operator11/1 -> Logical Operator4/1
  Relational Operator2/1 -> Logical Operator4/2
  Relational Operator10/1 -> Logical Operator3/1
  Relational Operator3/1 -> Logical Operator3/2
  Relational Operator9/1 -> Logical Operator2/1
  Relational Operator4/1 -> Logical Operator2/2
  Relational Operator8/1 -> Logical Operator1/1
  Relational Operator5/1 -> Logical Operator1/2
  Relational Operator/1 -> Logical Operator6/1
  Logical Operator/1 -> Logical Operator6/2
  Logical Operator5/1 -> Logical Operator7/1
  Logical Operator1/1 -> Logical Operator7/2
  Logical Operator4/1 -> Logical Operator8/1
  Logical Operator2/1 -> Logical Operator8/2
  Logical Operator6/1 -> Gain/1
  Logical Operator7/1 -> Gain1/1
  Logical Operator8/1 -> Gain2/1
  Logical Operator3/1 -> Gain3/1
  Gain3/1 -> Data Type Conversion3/1
  Gain2/1 -> Data Type Conversion2/1
  Gain1/1 -> Data Type Conversion1/1
  Gain/1 -> Data Type Conversion/1
  Data Type Conversion/1 -> Mux/1
  Data Type Conversion1/1 -> Mux/2
  Data Type Conversion2/1 -> Mux/3
  Data Type Conversion3/1 -> Mux/4
  Mux/1 -> V/1
  Fcn1/1 -> Relational Operator1/2, Relational Operator11/2
  Fcn3/1 -> Relational Operator9/2, Relational Operator3/2
  ramp/1 -> Relational Operator/1, Relational Operator12/1, Relational Operator1/1, Relational Operator11/1, Relational Operator2/1, Relational Operator10/1, Relational Operator3/1, Relational Operator9/1, Relational Operator4/1, Relational Operator8/1, Relational Operator5/1, Relational Operator7/1, Relational Operator6/1
  Fcn6/1 -> Relational Operator6/2
  Txy-07/1 -> Fcn/1, Fcn2/1, Fcn3/1, Fcn4/1, Fcn6/1, Fcn5/1, Fcn1/1
  Fcn2/1 -> Relational Operator10/2, Relational Operator2/2
  Fcn5/1 -> Relational Operator5/2, Relational Operator7/2
  Fcn4/1 -> Relational Operator8/2, Relational Operator4/2
  Fcn/1 -> Relational Operator12/2, Relational Operator/2

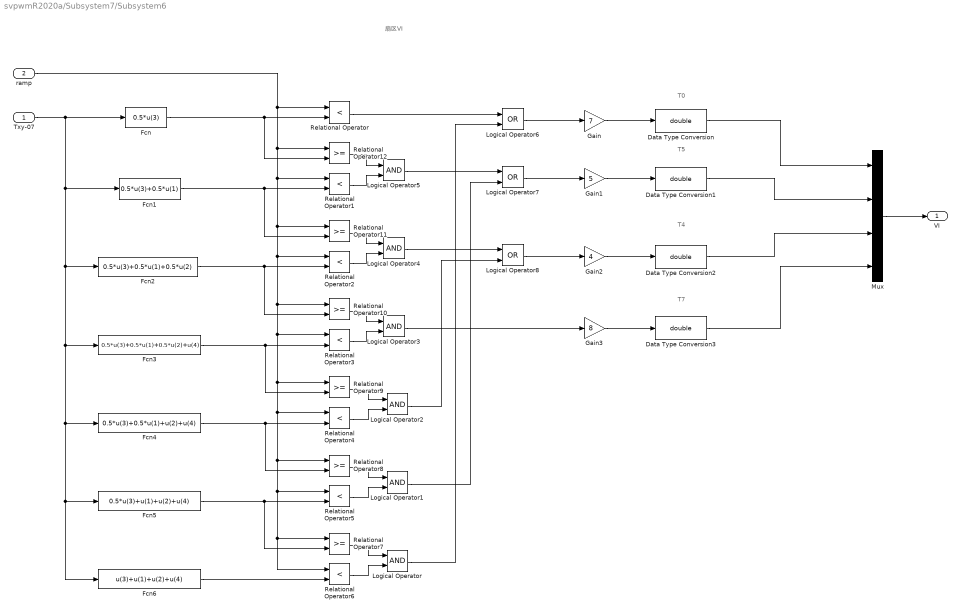
== system svpwmR2020a/Subsystem7/Subsystem6 ==
  note: T7
  note: 扇区VI
  note: T0
  note: T5
  note: T4
  Txy-07 : Inport
  ramp : Inport  Port=2
  Data Type Conversion{,1..3} (4 alike) : DataTypeConversion  OutDataTypeStr=double
  Fcn : Fcn  Expr=0.5*u(3)
  Fcn1 : Fcn  Expr=0.5*u(3)+0.5*u(1)
  Fcn2 : Fcn  Expr=0.5*u(3)+0.5*u(1)+0.5*u(2)
  Fcn3 : Fcn  Expr=0.5*u(3)+0.5*u(1)+0.5*u(2)+u(4)
  Fcn4 : Fcn  Expr=0.5*u(3)+0.5*u(1)+u(2)+u(4)
  Fcn5 : Fcn  Expr=0.5*u(3)+u(1)+u(2)+u(4)
  Fcn6 : Fcn  Expr=u(3)+u(1)+u(2)+u(4)
  Gain : Gain  Gain=7
  Gain1 : Gain  Gain=5
  Gain2 : Gain  Gain=4
  Gain3 : Gain  Gain=8
  Logical Operator{,1..5} (6 alike) : Logic  AllPortsSameDT=off  OutDataTypeStr=boolean
  Logical Operator6 : Logic  Operator=OR  AllPortsSameDT=off  OutDataTypeStr=boolean
  Logical Operator7 : Logic  Operator=OR  AllPortsSameDT=off  OutDataTypeStr=boolean
  Logical Operator8 : Logic  Operator=OR  AllPortsSameDT=off  OutDataTypeStr=boolean
  Mux : Mux
  Relational Operator{,1..6} (7 alike) : RelationalOperator  Operator=<  OutDataTypeStr=boolean  RndMeth=Simplest
  Relational Operator{7..12} (6 alike) : RelationalOperator  OutDataTypeStr=boolean  RndMeth=Simplest
  VI : Outport
  wires:
  Mux/1 -> VI/1
  Data Type Conversion3/1 -> Mux/4
  Data Type Conversion2/1 -> Mux/3
  Data Type Conversion1/1 -> Mux/2
  Data Type Conversion/1 -> Mux/1
  Gain/1 -> Data Type Conversion/1
  Gain1/1 -> Data Type Conversion1/1
  Gain2/1 -> Data Type Conversion2/1
  Gain3/1 -> Data Type Conversion3/1
  Logical Operator3/1 -> Gain3/1
  Logical Operator8/1 -> Gain2/1
  Logical Operator7/1 -> Gain1/1
  Logical Operator6/1 -> Gain/1
  Logical Operator2/1 -> Logical Operator8/2
  Logical Operator4/1 -> Logical Operator8/1
  Logical Operator1/1 -> Logical Operator7/2
  Logical Operator5/1 -> Logical Operator7/1
  Logical Operator/1 -> Logical Operator6/2
  Relational Operator/1 -> Logical Operator6/1
  Relational Operator5/1 -> Logical Operator1/2
  Relational Operator8/1 -> Logical Operator1/1
  Relational Operator4/1 -> Logical Operator2/2
  Relational Operator9/1 -> Logical Operator2/1
  Relational Operator3/1 -> Logical Operator3/2
  Relational Operator10/1 -> Logical Operator3/1
  Relational Operator2/1 -> Logical Operator4/2
  Relational Operator11/1 -> Logical Operator4/1
  Relational Operator1/1 -> Logical Operator5/2
  Relational Operator12/1 -> Logical Operator5/1
  Relational Operator6/1 -> Logical Operator/2
  Relational Operator7/1 -> Logical Operator/1
  Fcn1/1 -> Relational Operator11/2, Relational Operator1/2
  Fcn3/1 -> Relational Operator3/2, Relational Operator9/2
  ramp/1 -> Relational Operator/1, Relational Operator12/1, Relational Operator1/1, Relational Operator11/1, Relational Operator2/1, Relational Operator10/1, Relational Operator3/1, Relational Operator9/1, Relational Operator4/1, Relational Operator8/1, Relational Operator5/1, Relational Operator6/1, Relational Operator7/1
  Fcn6/1 -> Relational Operator6/2
  Txy-07/1 -> Fcn/1, Fcn2/1, Fcn3/1, Fcn4/1, Fcn6/1, Fcn5/1, Fcn1/1
  Fcn2/1 -> Relational Operator10/2, Relational Operator2/2
  Fcn5/1 -> Relational Operator5/2, Relational Operator7/2
  Fcn4/1 -> Relational Operator8/2, Relational Operator4/2
  Fcn/1 -> Relational Operator/2, Relational Operator12/2
